simulink model "Simulation_in_Simulink"  (R2021b)
settings: Solver=FixedStepAuto  StartTime=0.0  StopTime=10  FixedStep=0.02  RelTol=1e-3
(part 5 of 5)

== matlab function Simulation_in_Simulink/M ==
  data: theta input; M output
function M = fcn(theta)


t1=theta(1);
t2=theta(2);
t3=theta(3);
t4=theta(4);
t5=theta(5);
t6=theta(6);


a2=0.6129;
a3=0.5716; 
d4=0.16389; 
d5=0.1157; 
d6=0.0922;

M = [(49450651*cos(2*t2 + 2*t3 + 2*t4 - t5))/250000000000 - (37373*d5)/2500000 - (37373*d4)/1250000 - (1966511423*cos(2*t2 + 2*t3 + 2*t4 - 2*t5))/20000000000000 - (1966511423*cos(2*t2 + 2*t3 + 2*t4 + 2*t5))/20000000000000 + (53*cos(2*t2))/40 + (1966511423*cos(2*t5))/10000000000000 - (3534581023*cos(2*t2 + 2*t3 + 2*t4))/10000000000000 + (42783*cos(2*t2 + 2*t3))/62500 - (49450651*cos(2*t2 + 2*t3 + 2*t4 + t5))/250000000000 + (37373*d5*cos(2*t2 + 2*t3 + 2*t4))/2500000 - (957929*a2*sin(2*t2 + t3 + t4 - t5))/100000000 + (957929*a3*sin(2*t2 + 2*t3 + t4 + t5))/100000000 + (sin(t2 + t3 + t4)^2*sin(t5)^2)/2500 - (210469*a2*sin(2*t2 + t3 + t4))/50000000 - (957929*a2*sin(t3 + t4 - t5))/100000000 + (8247*a2^2*cos(2*t2))/1000 - (1967*d5^2*cos(2*t2 + 2*t3 + 2*t4))/2000 + (cos(t2 + t3 + t4)*cos(t6) - sin(t2 + t3 + t4)*cos(t5)*sin(t6))*((3*cos(t2 + t3 + t4)*cos(t6))/12500 - (3*sin(t2 + t3 + t4)*cos(t5)*sin(t6))/12500) + (cos(t2 + t3 + t4)*sin(t6) + sin(t2 + t3 + t4)*cos(t5)*cos(t6))*((11*cos(t2 + t3 + t4)*sin(t6))/50000 + (11*sin(t2 + t3 + t4)*cos(t5)*cos(t6))/50000) + (957929*d5*cos(2*t2 + 2*t3 + 2*t4 + t5))/100000000 - (210469*a2*sin(t3 + t4))/50000000 + (957929*a3*sin(t4 + t5))/100000000 - (957929*a3*sin(2*t2 + 2*t3 + t4 - t5))/100000000 + (1967*a3^2*cos(2*t2 + 2*t3))/1000 + (2041*a2*cos(t3))/625 + (957929*d4*cos(t5))/25000000 + (d6*(cos(t5)*sin(t1) + cos(t2 + t3 + t4)*cos(t1)*sin(t5)) - (873*cos(t5)*sin(t1))/50000 - (19*sin(t6)*(sin(t1)*sin(t5) - cos(t2 + t3 + t4)*cos(t1)*cos(t5)))/20000 + d4*sin(t1) - (873*cos(t2 + t3 + t4)*cos(t1)*sin(t5))/50000 + (19*sin(t2 + t3 + t4)*cos(t1)*cos(t6))/20000 + a3*cos(t2 + t3)*cos(t1) + a2*cos(t1)*cos(t2) - d5*sin(t2 + t3 + t4)*cos(t1))*((43*d6*(cos(t5)*sin(t1) + cos(t2 + t3 + t4)*cos(t1)*sin(t5)))/100 - (37539*cos(t5)*sin(t1))/5000000 - (817*sin(t6)*(sin(t1)*sin(t5) - cos(t2 + t3 + t4)*cos(t1)*cos(t5)))/2000000 + (43*d4*sin(t1))/100 - (37539*cos(t2 + t3 + t4)*cos(t1)*sin(t5))/5000000 + (817*sin(t2 + t3 + t4)*cos(t1)*cos(t6))/2000000 + (43*a3*cos(t2 + t3)*cos(t1))/100 + (43*a2*cos(t1)*cos(t2))/100 - (43*d5*sin(t2 + t3 + t4)*cos(t1))/100) - (210469*a3*sin(t4))/50000000 - (210469*a3*sin(2*t2 + 2*t3 + t4))/50000000 + (8247*a2^2)/1000 + (1967*a3^2)/1000 + (957929*a2*sin(2*t2 + t3 + t4 + t5))/100000000 + (1967*d4^2)/500 + (1967*d5^2)/2000 + (2041*a2*cos(2*t2 + t3))/625 - (957929*d5*cos(2*t2 + 2*t3 + 2*t4 - t5))/100000000 - (957929*a3*sin(t4 - t5))/100000000 + (957929*a2*sin(t3 + t4 + t5))/100000000 + ((19*sin(t6)*(cos(t1)*sin(t5) + cos(t2 + t3 + t4)*cos(t5)*sin(t1)))/20000 + (873*cos(t1)*cos(t5))/50000 - d6*(cos(t1)*cos(t5) - cos(t2 + t3 + t4)*sin(t1)*sin(t5)) - d4*cos(t1) - (873*cos(t2 + t3 + t4)*sin(t1)*sin(t5))/50000 + (19*sin(t2 + t3 + t4)*cos(t6)*sin(t1))/20000 + a3*cos(t2 + t3)*sin(t1) + a2*cos(t2)*sin(t1) - d5*sin(t2 + t3 + t4)*sin(t1))*((817*sin(t6)*(cos(t1)*sin(t5) + cos(t2 + t3 + t4)*cos(t5)*sin(t1)))/2000000 + (37539*cos(t1)*cos(t5))/5000000 - (43*d6*(cos(t1)*cos(t5) - cos(t2 + t3 + t4)*sin(t1)*sin(t5)))/100 - (43*d4*cos(t1))/100 - (37539*cos(t2 + t3 + t4)*sin(t1)*sin(t5))/5000000 + (817*sin(t2 + t3 + t4)*cos(t6)*sin(t1))/2000000 + (43*a3*cos(t2 + t3)*sin(t1))/100 + (43*a2*cos(t2)*sin(t1))/100 - (43*d5*sin(t2 + t3 + t4)*sin(t1))/100) - (1967*a3*d5*sin(t4))/1000 - (1967*a3*d5*sin(2*t2 + 2*t3 + t4))/1000 + (1967*a2*a3*cos(2*t2 + t3))/500 - (1967*a2*d5*sin(2*t2 + t3 + t4))/1000 - (1967*a2*d5*sin(t3 + t4))/1000 + (1967*a2*a3*cos(t3))/500 + 5654679353183/2000000000000, (49450651*cos(t2 + t3 + t4))/125000000000 - (713241*cos(t2 + t3 + t4 + t5 + t6))/400000000000 - (713241*cos(t2 + t3 + t4 + t5 - t6))/400000000000 - (713241*cos(t2 + t3 + t4 - t5 + t6))/400000000000 + (784477*cos(t2 + t3 + t4 + t5 - 2*t6))/320000000000 - (784477*cos(t2 + t3 + t4 + t5 + 2*t6))/320000000000 - (713241*cos(t2 + t3 + t4 - 2*t5 + t6))/400000000000 - (713241*cos(t2 + t3 + t4 + 2*t5 + t6))/400000000000 + (49450651*cos(t2 + t3 + t4 + t5))/250000000000 - (2041*sin(t2 + t3))/12500 - (713241*cos(t2 + t3 + t4 - t5 - t6))/400000000000 - (784477*cos(t2 + t3 + t4 - t5 - 2*t6))/320000000000 + (784477*cos(t2 + t3 + t4 - t5 + 2*t6))/320000000000 + (713241*cos(t2 + t3 + t4 - 2*t5 - t6))/400000000000 + (713241*cos(t2 + t3 + t4 + 2*t5 - t6))/400000000000 + (784477*cos(t2 + t3 + t4 - 2*t5 - 2*t6))/640000000000 + (784477*cos(t2 + t3 + t4 - 2*t5 + 2*t6))/640000000000 - (784477*cos(t2 + t3 + t4 + 2*t5 - 2*t6))/640000000000 - (784477*cos(t2 + t3 + t4 + 2*t5 + 2*t6))/640000000000 - (1237*sin(t2))/1250 + (49450651*cos(t2 + t3 + t4 - t5))/250000000000 - (7474967197*cos(t2 + t3 + t4 - 2*t5))/40000000000000 + (7474967197*cos(t2 + t3 + t4 + 2*t5))/40000000000000 - (43*d6^2*cos(t2 + t3 + t4 - 2*t5))/400 + (43*d6^2*cos(t2 + t3 + t4 + 2*t5))/400 - (817*a3*sin(t2 + t3 - t5 - t6))/8000000 - (817*d4*cos(t2 + t3 + t4 + t5 - t6))/8000000 + (817*d4*cos(t2 + t3 + t4 - t5 + t6))/8000000 + (817*d5*cos(t2 + t3 + t4 + t5 - t6))/8000000 + (817*d5*cos(t2 + t3 + t4 - t5 + t6))/8000000 + (817*d6*cos(t2 + t3 + t4 + t5 - t6))/8000000 + (817*d6*cos(t2 + t3 + t4 - t5 + t6))/8000000 + (817*d6*cos(t2 + t3 + t4 - 2*t5 + t6))/8000000 + (817*d6*cos(t2 + t3 + t4 + 2*t5 + t6))/8000000 - (582539*a3*sin(t2 + t3 - t5))/100000000 + (817*a2*sin(t2 + t5 - t6))/8000000 + (817*a2*sin(t2 - t5 + t6))/8000000 + (817*a2*sin(t5 - t2 + t6))/8000000 + (582539*d4*cos(t2 + t3 + t4 + t5))/100000000 + (817*d4*cos(t2 + t3 + t4 + t6))/4000000 - (582539*d5*cos(t2 + t3 + t4 + t5))/100000000 - (817*a3*sin(t2 + t3 + t5 + t6))/8000000 + (37373*a3*sin(t2 + t3))/2500000 - (582539*a2*sin(t2 + t5))/100000000 - (817*d4*cos(t2 + t3 + t4 - t5 - t6))/8000000 - (817*d5*cos(t2 + t3 + t4 - t5 - t6))/8000000 + (817*d6*cos(t2 + t3 + t4 - t5 - t6))/8000000 - (817*d6*cos(t2 + t3 + t4 - 2*t5 - t6))/8000000 - (817*d6*cos(t2 + t3 + t4 + 2*t5 - t6))/8000000 - (1532627*a2*sin(t2))/2500000 - (582539*d4*cos(t2 + t3 + t4 - t5))/100000000 + (817*d4*cos(t2 + t3 + t4 - t6))/4000000 - (582539*d5*cos(t2 + t3 + t4 - t5))/100000000 + (37539*d6*cos(t2 + t3 + t4 - 2*t5))/10000000 - (37539*d6*cos(t2 + t3 + t4 + 2*t5))/10000000 + (817*a3*sin(t2 + t3 + t5 - t6))/8000000 + (817*a3*sin(t2 + t3 - t5 + t6))/8000000 + (817*d4*cos(t2 + t3 + t4 + t5 + t6))/8000000 - (817*d5*cos(t2 + t3 + t4 + t5 + t6))/8000000 + (817*d6*cos(t2 + t3 + t4 + t5 + t6))/8000000 - (582539*a2*sin(t2 - t5))/100000000 - (210469*d4*cos(t2 + t3 + t4))/50000000 - (582539*a3*sin(t2 + t3 + t5))/100000000 - (817*a2*sin(t2 + t5 + t6))/8000000 - (1091*a2*d4*sin(t2))/250 - (43*d4*d6*cos(t2 + t3 + t4 - t5))/200 - (43*d5*d6*cos(t2 + t3 + t4 - t5))/200 - (43*a2*d6*sin(t2 - t5))/200 - (2397*d4*d5*cos(t2 + t3 + t4))/1000 - (43*a3*d6*sin(t2 + t3 + t5))/200 - (43*a3*d6*sin(t2 + t3 - t5))/200 + (43*d4*d6*cos(t2 + t3 + t4 + t5))/200 - (43*d5*d6*cos(t2 + t3 + t4 + t5))/200 - (1091*a3*d4*sin(t2 + t3))/250 - (43*a2*d6*sin(t2 + t5))/200, (49450651*cos(t2 + t3 + t4))/125000000000 - (713241*cos(t2 + t3 + t4 + t5 + t6))/400000000000 - (713241*cos(t2 + t3 + t4 + t5 - t6))/400000000000 - (713241*cos(t2 + t3 + t4 - t5 + t6))/400000000000 + (784477*cos(t2 + t3 + t4 + t5 - 2*t6))/320000000000 - (784477*cos(t2 + t3 + t4 + t5 + 2*t6))/320000000000 - (713241*cos(t2 + t3 + t4 - 2*t5 + t6))/400000000000 - (713241*cos(t2 + t3 + t4 + 2*t5 + t6))/400000000000 + (49450651*cos(t2 + t3 + t4 + t5))/250000000000 - (2041*sin(t2 + t3))/12500 - (713241*cos(t2 + t3 + t4 - t5 - t6))/400000000000 - (784477*cos(t2 + t3 + t4 - t5 - 2*t6))/320000000000 + (784477*cos(t2 + t3 + t4 - t5 + 2*t6))/320000000000 + (713241*cos(t2 + t3 + t4 - 2*t5 - t6))/400000000000 + (713241*cos(t2 + t3 + t4 + 2*t5 - t6))/400000000000 + (784477*cos(t2 + t3 + t4 - 2*t5 - 2*t6))/640000000000 + (784477*cos(t2 + t3 + t4 - 2*t5 + 2*t6))/640000000000 - (784477*cos(t2 + t3 + t4 + 2*t5 - 2*t6))/640000000000 - (784477*cos(t2 + t3 + t4 + 2*t5 + 2*t6))/640000000000 + (49450651*cos(t2 + t3 + t4 - t5))/250000000000 - (7474967197*cos(t2 + t3 + t4 - 2*t5))/40000000000000 + (7474967197*cos(t2 + t3 + t4 + 2*t5))/40000000000000 - (43*d6^2*cos(t2 + t3 + t4 - 2*t5))/400 + (43*d6^2*cos(t2 + t3 + t4 + 2*t5))/400 - (817*a3*sin(t2 + t3 - t5 - t6))/8000000 - (817*d4*cos(t2 + t3 + t4 + t5 - t6))/8000000 + (817*d4*cos(t2 + t3 + t4 - t5 + t6))/8000000 + (817*d5*cos(t2 + t3 + t4 + t5 - t6))/8000000 + (817*d5*cos(t2 + t3 + t4 - t5 + t6))/8000000 + (817*d6*cos(t2 + t3 + t4 + t5 - t6))/8000000 + (817*d6*cos(t2 + t3 + t4 - t5 + t6))/8000000 + (817*d6*cos(t2 + t3 + t4 - 2*t5 + t6))/8000000 + (817*d6*cos(t2 + t3 + t4 + 2*t5 + t6))/8000000 - (582539*a3*sin(t2 + t3 - t5))/100000000 + (582539*d4*cos(t2 + t3 + t4 + t5))/100000000 + (817*d4*cos(t2 + t3 + t4 + t6))/4000000 - (582539*d5*cos(t2 + t3 + t4 + t5))/100000000 - (817*a3*sin(t2 + t3 + t5 + t6))/8000000 + (37373*a3*sin(t2 + t3))/2500000 - (817*d4*cos(t2 + t3 + t4 - t5 - t6))/8000000 - (817*d5*cos(t2 + t3 + t4 - t5 - t6))/8000000 + (817*d6*cos(t2 + t3 + t4 - t5 - t6))/8000000 - (817*d6*cos(t2 + t3 + t4 - 2*t5 - t6))/8000000 - (817*d6*cos(t2 + t3 + t4 + 2*t5 - t6))/8000000 - (582539*d4*cos(t2 + t3 + t4 - t5))/100000000 + (817*d4*cos(t2 + t3 + t4 - t6))/4000000 - (582539*d5*cos(t2 + t3 + t4 - t5))/100000000 + (37539*d6*cos(t2 + t3 + t4 - 2*t5))/10000000 - (37539*d6*cos(t2 + t3 + t4 + 2*t5))/10000000 + (817*a3*sin(t2 + t3 + t5 - t6))/8000000 + (817*a3*sin(t2 + t3 - t5 + t6))/8000000 + (817*d4*cos(t2 + t3 + t4 + t5 + t6))/8000000 - (817*d5*cos(t2 + t3 + t4 + t5 + t6))/8000000 + (817*d6*cos(t2 + t3 + t4 + t5 + t6))/8000000 - (210469*d4*cos(t2 + t3 + t4))/50000000 - (582539*a3*sin(t2 + t3 + t5))/100000000 - (43*d4*d6*cos(t2 + t3 + t4 - t5))/200 - (43*d5*d6*cos(t2 + t3 + t4 - t5))/200 - (2397*d4*d5*cos(t2 + t3 + t4))/1000 - (43*a3*d6*sin(t2 + t3 + t5))/200 - (43*a3*d6*sin(t2 + t3 - t5))/200 + (43*d4*d6*cos(t2 + t3 + t4 + t5))/200 - (43*d5*d6*cos(t2 + t3 + t4 + t5))/200 - (1091*a3*d4*sin(t2 + t3))/250, (49450651*cos(t2 + t3 + t4))/125000000000 - (713241*cos(t2 + t3 + t4 + t5 + t6))/400000000000 - (713241*cos(t2 + t3 + t4 + t5 - t6))/400000000000 - (713241*cos(t2 + t3 + t4 - t5 + t6))/400000000000 + (784477*cos(t2 + t3 + t4 + t5 - 2*t6))/320000000000 - (784477*cos(t2 + t3 + t4 + t5 + 2*t6))/320000000000 - (713241*cos(t2 + t3 + t4 - 2*t5 + t6))/400000000000 - (713241*cos(t2 + t3 + t4 + 2*t5 + t6))/400000000000 + (49450651*cos(t2 + t3 + t4 + t5))/250000000000 - (713241*cos(t2 + t3 + t4 - t5 - t6))/400000000000 - (784477*cos(t2 + t3 + t4 - t5 - 2*t6))/320000000000 + (784477*cos(t2 + t3 + t4 - t5 + 2*t6))/320000000000 + (713241*cos(t2 + t3 + t4 - 2*t5 - t6))/400000000000 + (713241*cos(t2 + t3 + t4 + 2*t5 - t6))/400000000000 + (784477*cos(t2 + t3 + t4 - 2*t5 - 2*t6))/640000000000 + (784477*cos(t2 + t3 + t4 - 2*t5 + 2*t6))/640000000000 - (784477*cos(t2 + t3 + t4 + 2*t5 - 2*t6))/640000000000 - (784477*cos(t2 + t3 + t4 + 2*t5 + 2*t6))/640000000000 + (49450651*cos(t2 + t3 + t4 - t5))/250000000000 - (7474967197*cos(t2 + t3 + t4 - 2*t5))/40000000000000 + (7474967197*cos(t2 + t3 + t4 + 2*t5))/40000000000000 - (43*d6^2*cos(t2 + t3 + t4 - 2*t5))/400 + (43*d6^2*cos(t2 + t3 + t4 + 2*t5))/400 - (817*d4*cos(t2 + t3 + t4 + t5 - t6))/8000000 + (817*d4*cos(t2 + t3 + t4 - t5 + t6))/8000000 + (817*d5*cos(t2 + t3 + t4 + t5 - t6))/8000000 + (817*d5*cos(t2 + t3 + t4 - t5 + t6))/8000000 + (817*d6*cos(t2 + t3 + t4 + t5 - t6))/8000000 + (817*d6*cos(t2 + t3 + t4 - t5 + t6))/8000000 + (817*d6*cos(t2 + t3 + t4 - 2*t5 + t6))/8000000 + (817*d6*cos(t2 + t3 + t4 + 2*t5 + t6))/8000000 + (582539*d4*cos(t2 + t3 + t4 + t5))/100000000 + (817*d4*cos(t2 + t3 + t4 + t6))/4000000 - (582539*d5*cos(t2 + t3 + t4 + t5))/100000000 - (817*d4*cos(t2 + t3 + t4 - t5 - t6))/8000000 - (817*d5*cos(t2 + t3 + t4 - t5 - t6))/8000000 + (817*d6*cos(t2 + t3 + t4 - t5 - t6))/8000000 - (817*d6*cos(t2 + t3 + t4 - 2*t5 - t6))/8000000 - (817*d6*cos(t2 + t3 + t4 + 2*t5 - t6))/8000000 - (582539*d4*cos(t2 + t3 + t4 - t5))/100000000 + (817*d4*cos(t2 + t3 + t4 - t6))/4000000 - (582539*d5*cos(t2 + t3 + t4 - t5))/100000000 + (37539*d6*cos(t2 + t3 + t4 - 2*t5))/10000000 - (37539*d6*cos(t2 + t3 + t4 + 2*t5))/10000000 + (817*d4*cos(t2 + t3 + t4 + t5 + t6))/8000000 - (817*d5*cos(t2 + t3 + t4 + t5 + t6))/8000000 + (817*d6*cos(t2 + t3 + t4 + t5 + t6))/8000000 - (210469*d4*cos(t2 + t3 + t4))/50000000 - (43*d4*d6*cos(t2 + t3 + t4 - t5))/200 - (43*d5*d6*cos(t2 + t3 + t4 - t5))/200 - (2397*d4*d5*cos(t2 + t3 + t4))/1000 + (43*d4*d6*cos(t2 + t3 + t4 + t5))/200 - (43*d5*d6*cos(t2 + t3 + t4 + t5))/200, (713241*cos(t2 + t3 + t4 + t5 + t6))/400000000000 + (33478847947*cos(t2 + t3 + t4))/10000000000000 + (713241*cos(t2 + t3 + t4 + t5 - t6))/400000000000 - (713241*cos(t2 + t3 + t4 - t5 + t6))/400000000000 - (784477*cos(t2 + t3 + t4 + t5 - 2*t6))/320000000000 + (784477*cos(t2 + t3 + t4 + t5 + 2*t6))/320000000000 - (49450651*cos(t2 + t3 + t4 + t5))/250000000000 - (713241*cos(t2 + t3 + t4 - t5 - t6))/400000000000 - (784477*cos(t2 + t3 + t4 - t5 - 2*t6))/320000000000 + (784477*cos(t2 + t3 + t4 - t5 + 2*t6))/320000000000 + (49450651*cos(t2 + t3 + t4 - t5))/250000000000 + (784477*cos(t2 + t3 + t4 - 2*t6))/160000000000 + (784477*cos(t2 + t3 + t4 + 2*t6))/160000000000 - (817*a3*sin(t2 + t3 - t5 - t6))/8000000 - (817*d4*cos(t2 + t3 + t4 + t5 - t6))/8000000 - (817*d4*cos(t2 + t3 + t4 - t5 + t6))/8000000 - (817*d5*cos(t2 + t3 + t4 + t5 - t6))/8000000 + (817*d5*cos(t2 + t3 + t4 - t5 + t6))/8000000 - (817*d6*cos(t2 + t3 + t4 + t5 - t6))/8000000 + (817*d6*cos(t2 + t3 + t4 - t5 + t6))/8000000 + (43*d6^2*cos(t2 + t3 + t4))/100 - (582539*a3*sin(t2 + t3 - t5))/100000000 - (817*a2*sin(t2 + t5 - t6))/8000000 + (817*a2*sin(t2 - t5 + t6))/8000000 + (817*a2*sin(t5 - t2 + t6))/8000000 + (582539*d4*cos(t2 + t3 + t4 + t5))/100000000 + (582539*d5*cos(t2 + t3 + t4 + t5))/100000000 + (817*a3*sin(t2 + t3 + t5 + t6))/8000000 + (582539*a2*sin(t2 + t5))/100000000 + (817*d4*cos(t2 + t3 + t4 - t5 - t6))/8000000 - (817*d5*cos(t2 + t3 + t4 - t5 - t6))/8000000 + (817*d6*cos(t2 + t3 + t4 - t5 - t6))/8000000 + (582539*d4*cos(t2 + t3 + t4 - t5))/100000000 - (582539*d5*cos(t2 + t3 + t4 - t5))/100000000 - (817*a3*sin(t2 + t3 + t5 - t6))/8000000 + (817*a3*sin(t2 + t3 - t5 + t6))/8000000 + (817*d4*cos(t2 + t3 + t4 + t5 + t6))/8000000 + (817*d5*cos(t2 + t3 + t4 + t5 + t6))/8000000 - (817*d6*cos(t2 + t3 + t4 + t5 + t6))/8000000 - (582539*a2*sin(t2 - t5))/100000000 - (37539*d6*cos(t2 + t3 + t4))/2500000 + (582539*a3*sin(t2 + t3 + t5))/100000000 + (817*a2*sin(t2 + t5 + t6))/8000000 + (43*d4*d6*cos(t2 + t3 + t4 - t5))/200 - (43*d5*d6*cos(t2 + t3 + t4 - t5))/200 - (43*a2*d6*sin(t2 - t5))/200 + (43*a3*d6*sin(t2 + t3 + t5))/200 - (43*a3*d6*sin(t2 + t3 - t5))/200 + (43*d4*d6*cos(t2 + t3 + t4 + t5))/200 + (43*d5*d6*cos(t2 + t3 + t4 + t5))/200 + (43*a2*d6*sin(t2 + t5))/200, (817*a2*cos(t2)*cos(t6)*sin(t5))/2000000 - (713241*cos(t2)*cos(t3)*cos(t4)*cos(t6))/100000000000 + (16015523*cos(t2)*cos(t3)*sin(t4)*sin(t5))/40000000000 + (16015523*cos(t2)*cos(t4)*sin(t3)*sin(t5))/40000000000 + (16015523*cos(t3)*cos(t4)*sin(t2)*sin(t5))/40000000000 + (713241*cos(t2)*cos(t6)*sin(t3)*sin(t4))/100000000000 + (713241*cos(t3)*cos(t6)*sin(t2)*sin(t4))/100000000000 + (713241*cos(t4)*cos(t6)*sin(t2)*sin(t3))/100000000000 - (16015523*sin(t2)*sin(t3)*sin(t4)*sin(t5))/40000000000 + (817*d6*cos(t2)*cos(t3)*cos(t4)*cos(t6))/2000000 + (817*a3*cos(t2)*cos(t3)*cos(t6)*sin(t5))/2000000 - (817*d4*cos(t2)*cos(t3)*sin(t4)*sin(t6))/2000000 - (817*d4*cos(t2)*cos(t4)*sin(t3)*sin(t6))/2000000 - (817*d4*cos(t3)*cos(t4)*sin(t2)*sin(t6))/2000000 - (817*d6*cos(t2)*cos(t6)*sin(t3)*sin(t4))/2000000 - (817*d6*cos(t3)*cos(t6)*sin(t2)*sin(t4))/2000000 - (817*d6*cos(t4)*cos(t6)*sin(t2)*sin(t3))/2000000 - (817*a3*cos(t6)*sin(t2)*sin(t3)*sin(t5))/2000000 + (817*d4*sin(t2)*sin(t3)*sin(t4)*sin(t6))/2000000 + (713241*cos(t2)*cos(t3)*cos(t5)*sin(t4)*sin(t6))/100000000000 + (713241*cos(t2)*cos(t4)*cos(t5)*sin(t3)*sin(t6))/100000000000 + (713241*cos(t3)*cos(t4)*cos(t5)*sin(t2)*sin(t6))/100000000000 - (713241*cos(t5)*sin(t2)*sin(t3)*sin(t4)*sin(t6))/100000000000 - (817*d4*cos(t2)*cos(t5)*cos(t6)*sin(t3)*sin(t4))/2000000 - (817*d4*cos(t3)*cos(t5)*cos(t6)*sin(t2)*sin(t4))/2000000 - (817*d4*cos(t4)*cos(t5)*cos(t6)*sin(t2)*sin(t3))/2000000 - (817*d5*cos(t2)*cos(t3)*cos(t6)*sin(t4)*sin(t5))/2000000 - (817*d5*cos(t2)*cos(t4)*cos(t6)*sin(t3)*sin(t5))/2000000 - (817*d5*cos(t3)*cos(t4)*cos(t6)*sin(t2)*sin(t5))/2000000 - (817*d6*cos(t2)*cos(t3)*cos(t5)*sin(t4)*sin(t6))/2000000 - (817*d6*cos(t2)*cos(t4)*cos(t5)*sin(t3)*sin(t6))/2000000 - (817*d6*cos(t3)*cos(t4)*cos(t5)*sin(t2)*sin(t6))/2000000 + (817*d5*cos(t6)*sin(t2)*sin(t3)*sin(t4)*sin(t5))/2000000 + (817*d6*cos(t5)*sin(t2)*sin(t3)*sin(t4)*sin(t6))/2000000 + (817*d4*cos(t2)*cos(t3)*cos(t4)*cos(t5)*cos(t6))/2000000;
                                                                                                              (49450651*cos(t2 + t3 + t4))/125000000000 - (713241*cos(t2 + t3 + t4 + t5 + t6))/400000000000 - (713241*cos(t2 + t3 + t4 + t5 - t6))/400000000000 - (713241*cos(t2 + t3 + t4 - t5 + t6))/400000000000 + (784477*cos(t2 + t3 + t4 + t5 - 2*t6))/320000000000 - (784477*cos(t2 + t3 + t4 + t5 + 2*t6))/320000000000 - (713241*cos(t2 + t3 + t4 - 2*t5 + t6))/400000000000 - (713241*cos(t2 + t3 + t4 + 2*t5 + t6))/400000000000 + (49450651*cos(t2 + t3 + t4 + t5))/250000000000 - (2041*sin(t2 + t3))/12500 - (713241*cos(t2 + t3 + t4 - t5 - t6))/400000000000 - (784477*cos(t2 + t3 + t4 - t5 - 2*t6))/320000000000 + (784477*cos(t2 + t3 + t4 - t5 + 2*t6))/320000000000 + (713241*cos(t2 + t3 + t4 - 2*t5 - t6))/400000000000 + (713241*cos(t2 + t3 + t4 + 2*t5 - t6))/400000000000 + (784477*cos(t2 + t3 + t4 - 2*t5 - 2*t6))/640000000000 + (784477*cos(t2 + t3 + t4 - 2*t5 + 2*t6))/640000000000 - (784477*cos(t2 + t3 + t4 + 2*t5 - 2*t6))/640000000000 - (784477*cos(t2 + t3 + t4 + 2*t5 + 2*t6))/640000000000 - (1237*sin(t2))/1250 + (49450651*cos(t2 + t3 + t4 - t5))/250000000000 - (7474967197*cos(t2 + t3 + t4 - 2*t5))/40000000000000 + (7474967197*cos(t2 + t3 + t4 + 2*t5))/40000000000000 - (43*d6^2*cos(t2 + t3 + t4 - 2*t5))/400 + (43*d6^2*cos(t2 + t3 + t4 + 2*t5))/400 - (817*a3*sin(t2 + t3 - t5 - t6))/8000000 - (817*d4*cos(t2 + t3 + t4 + t5 - t6))/8000000 + (817*d4*cos(t2 + t3 + t4 - t5 + t6))/8000000 + (817*d5*cos(t2 + t3 + t4 + t5 - t6))/8000000 + (817*d5*cos(t2 + t3 + t4 - t5 + t6))/8000000 + (817*d6*cos(t2 + t3 + t4 + t5 - t6))/8000000 + (817*d6*cos(t2 + t3 + t4 - t5 + t6))/8000000 + (817*d6*cos(t2 + t3 + t4 - 2*t5 + t6))/8000000 + (817*d6*cos(t2 + t3 + t4 + 2*t5 + t6))/8000000 - (582539*a3*sin(t2 + t3 - t5))/100000000 + (817*a2*sin(t2 + t5 - t6))/8000000 + (817*a2*sin(t2 - t5 + t6))/8000000 + (817*a2*sin(t5 - t2 + t6))/8000000 + (582539*d4*cos(t2 + t3 + t4 + t5))/100000000 + (817*d4*cos(t2 + t3 + t4 + t6))/4000000 - (582539*d5*cos(t2 + t3 + t4 + t5))/100000000 - (817*a3*sin(t2 + t3 + t5 + t6))/8000000 + (37373*a3*sin(t2 + t3))/2500000 - (582539*a2*sin(t2 + t5))/100000000 - (817*d4*cos(t2 + t3 + t4 - t5 - t6))/8000000 - (817*d5*cos(t2 + t3 + t4 - t5 - t6))/8000000 + (817*d6*cos(t2 + t3 + t4 - t5 - t6))/8000000 - (817*d6*cos(t2 + t3 + t4 - 2*t5 - t6))/8000000 - (817*d6*cos(t2 + t3 + t4 + 2*t5 - t6))/8000000 - (1532627*a2*sin(t2))/2500000 - (582539*d4*cos(t2 + t3 + t4 - t5))/100000000 + (817*d4*cos(t2 + t3 + t4 - t6))/4000000 - (582539*d5*cos(t2 + t3 + t4 - t5))/100000000 + (37539*d6*cos(t2 + t3 + t4 - 2*t5))/10000000 - (37539*d6*cos(t2 + t3 + t4 + 2*t5))/10000000 + (817*a3*sin(t2 + t3 + t5 - t6))/8000000 + (817*a3*sin(t2 + t3 - t5 + t6))/8000000 + (817*d4*cos(t2 + t3 + t4 + t5 + t6))/8000000 - (817*d5*cos(t2 + t3 + t4 + t5 + t6))/8000000 + (817*d6*cos(t2 + t3 + t4 + t5 + t6))/8000000 - (582539*a2*sin(t2 - t5))/100000000 - (210469*d4*cos(t2 + t3 + t4))/50000000 - (582539*a3*sin(t2 + t3 + t5))/100000000 - (817*a2*sin(t2 + t5 + t6))/8000000 - (1091*a2*d4*sin(t2))/250 - (43*d4*d6*cos(t2 + t3 + t4 - t5))/200 - (43*d5*d6*cos(t2 + t3 + t4 - t5))/200 - (43*a2*d6*sin(t2 - t5))/200 - (2397*d4*d5*cos(t2 + t3 + t4))/1000 - (43*a3*d6*sin(t2 + t3 + t5))/200 - (43*a3*d6*sin(t2 + t3 - t5))/200 + (43*d4*d6*cos(t2 + t3 + t4 + t5))/200 - (43*d5*d6*cos(t2 + t3 + t4 + t5))/200 - (1091*a3*d4*sin(t2 + t3))/250 - (43*a2*d6*sin(t2 + t5))/200,                                                                                                                                                                                                                                                                                                                                                                                                                                                                                                                                                                                                                                                                                                                                                                                                                                                                                                                                                                                                                                                                                                                                                                                                                                                                                                                                                                                                                                                                                                                                                                                                                                                                                                                                                                                                                                                                                                                                                                                                                                                                                                                                                                                                                               (4082*a2*cos(t3))/625 - (37539*d6)/2500000 - (3786513411*cos(t5)^2)/5000000000000 - (784477*cos(t6)^2)/40000000000 - (43*d6^2*cos(t5)^2)/100 - (37373*d5)/1250000 - (817*d5*cos(t6))/1000000 - (210469*a3*sin(t4))/25000000 + (4231*a2^2)/250 + (1091*a3^2)/250 + (2397*d5^2)/1000 + (43*d6^2)/100 + (784477*cos(t5)^2*cos(t6)^2)/40000000000 + (37539*d6*cos(t5)^2)/2500000 - (713241*cos(t5)*sin(t5)*sin(t6))/50000000000 - (2397*a3*d5*sin(t4))/500 - (210469*a2*cos(t3)*sin(t4))/25000000 - (210469*a2*cos(t4)*sin(t3))/25000000 + (582539*a3*cos(t4)*sin(t5))/25000000 + (817*a3*cos(t6)*sin(t4))/1000000 + (1091*a2*a3*cos(t3))/125 + (582539*a2*cos(t3)*cos(t4)*sin(t5))/25000000 + (817*a2*cos(t3)*cos(t6)*sin(t4))/1000000 + (817*a2*cos(t4)*cos(t6)*sin(t3))/1000000 + (817*a3*cos(t4)*cos(t5)*sin(t6))/1000000 + (817*d6*cos(t5)*sin(t5)*sin(t6))/1000000 - (582539*a2*sin(t3)*sin(t4)*sin(t5))/25000000 - (2397*a2*d5*cos(t3)*sin(t4))/500 - (2397*a2*d5*cos(t4)*sin(t3))/500 + (43*a3*d6*cos(t4)*sin(t5))/50 + (817*a2*cos(t3)*cos(t4)*cos(t5)*sin(t6))/1000000 - (817*a2*cos(t5)*sin(t3)*sin(t4)*sin(t6))/1000000 + (43*a2*d6*cos(t3)*cos(t4)*sin(t5))/50 - (43*a2*d6*sin(t3)*sin(t4)*sin(t5))/50 + 2553571193279/625000000000,                                                                                                                                                                                                                                                                                                                                                                                                                                                                                                                                                                                                                                                                                                                                                                                                                                                                                                                                                                                                                                                                                                                                                                                                                                                                                                                                                                                                                                                                                                                                                                                                                                                                                                                                                                                                                                                                    (2041*a2*cos(t3))/625 - (37539*d6)/2500000 - (3786513411*cos(t5)^2)/5000000000000 - (784477*cos(t6)^2)/40000000000 - (43*d6^2*cos(t5)^2)/100 - (37373*d5)/1250000 - (817*d5*cos(t6))/1000000 - (210469*a3*sin(t4))/25000000 + (1091*a3^2)/250 + (2397*d5^2)/1000 + (43*d6^2)/100 + (784477*cos(t5)^2*cos(t6)^2)/40000000000 + (37539*d6*cos(t5)^2)/2500000 - (713241*cos(t5)*sin(t5)*sin(t6))/50000000000 - (2397*a3*d5*sin(t4))/500 - (210469*a2*cos(t3)*sin(t4))/50000000 - (210469*a2*cos(t4)*sin(t3))/50000000 + (582539*a3*cos(t4)*sin(t5))/25000000 + (817*a3*cos(t6)*sin(t4))/1000000 + (1091*a2*a3*cos(t3))/250 + (582539*a2*cos(t3)*cos(t4)*sin(t5))/50000000 + (817*a2*cos(t3)*cos(t6)*sin(t4))/2000000 + (817*a2*cos(t4)*cos(t6)*sin(t3))/2000000 + (817*a3*cos(t4)*cos(t5)*sin(t6))/1000000 + (817*d6*cos(t5)*sin(t5)*sin(t6))/1000000 - (582539*a2*sin(t3)*sin(t4)*sin(t5))/50000000 - (2397*a2*d5*cos(t3)*sin(t4))/1000 - (2397*a2*d5*cos(t4)*sin(t3))/1000 + (43*a3*d6*cos(t4)*sin(t5))/50 + (817*a2*cos(t3)*cos(t4)*cos(t5)*sin(t6))/2000000 - (817*a2*cos(t5)*sin(t3)*sin(t4)*sin(t6))/2000000 + (43*a2*d6*cos(t3)*cos(t4)*sin(t5))/100 - (43*a2*d6*sin(t3)*sin(t4)*sin(t5))/100 + 872321193279/625000000000,                                                                                                                                                                                                                                                                                                                                                                                                                                                                                                                                                                                                                                                                                                                                                                                                                                                                                                                                                                                                                                                                                                                                                                                                                                                                                                                                                                                                                                                                                                         (2397*d5^2)/1000 - (37539*d6)/2500000 - (3786513411*cos(t5)^2)/5000000000000 - (784477*cos(t6)^2)/40000000000 - (43*d6^2*cos(t5)^2)/100 - (817*d5*cos(t6))/1000000 - (210469*a3*sin(t4))/50000000 - (37373*d5)/1250000 + (43*d6^2)/100 + (784477*cos(t5)^2*cos(t6)^2)/40000000000 + (37539*d6*cos(t5)^2)/2500000 - (713241*cos(t5)*sin(t5)*sin(t6))/50000000000 - (2397*a3*d5*sin(t4))/1000 - (210469*a2*cos(t3)*sin(t4))/50000000 - (210469*a2*cos(t4)*sin(t3))/50000000 + (582539*a3*cos(t4)*sin(t5))/50000000 + (817*a3*cos(t6)*sin(t4))/2000000 + (582539*a2*cos(t3)*cos(t4)*sin(t5))/50000000 + (817*a2*cos(t3)*cos(t6)*sin(t4))/2000000 + (817*a2*cos(t4)*cos(t6)*sin(t3))/2000000 + (817*a3*cos(t4)*cos(t5)*sin(t6))/2000000 + (817*d6*cos(t5)*sin(t5)*sin(t6))/1000000 - (582539*a2*sin(t3)*sin(t4)*sin(t5))/50000000 - (2397*a2*d5*cos(t3)*sin(t4))/1000 - (2397*a2*d5*cos(t4)*sin(t3))/1000 + (43*a3*d6*cos(t4)*sin(t5))/100 + (817*a2*cos(t3)*cos(t4)*cos(t5)*sin(t6))/2000000 - (817*a2*cos(t5)*sin(t3)*sin(t4)*sin(t6))/2000000 + (43*a2*d6*cos(t3)*cos(t4)*sin(t5))/100 - (43*a2*d6*sin(t3)*sin(t4)*sin(t5))/100 + 4161193279/625000000000,                                                                                                                                                                                                                                                                                                                                                                                                                                                                                                                                                                                                                                                                                                                                                                                                                                                                                                                                                                                                                                                                                                                                                                                                                                                                                                                                                                                                                                                                                                                                                                                                                                                                                   (49450651*cos(t5))/125000000000 - (713241*cos(t5)*cos(t6))/100000000000 - (582539*d5*cos(t5))/50000000 + (784477*cos(t6)*sin(t5)*sin(t6))/40000000000 + (817*d6*cos(t5)*cos(t6))/2000000 + (582539*a3*cos(t5)*sin(t4))/50000000 + (817*d5*sin(t5)*sin(t6))/2000000 - (43*d5*d6*cos(t5))/100 + (582539*a2*cos(t3)*cos(t5)*sin(t4))/50000000 + (582539*a2*cos(t4)*cos(t5)*sin(t3))/50000000 - (817*a3*sin(t4)*sin(t5)*sin(t6))/2000000 + (43*a3*d6*cos(t5)*sin(t4))/100 - (817*a2*cos(t3)*sin(t4)*sin(t5)*sin(t6))/2000000 - (817*a2*cos(t4)*sin(t3)*sin(t5)*sin(t6))/2000000 + (43*a2*d6*cos(t3)*cos(t5)*sin(t4))/100 + (43*a2*d6*cos(t4)*cos(t5)*sin(t3))/100,                                                                                                                                                                                                                                                                                                                                                                                                                                                                                                                                                                                                                                                                                                                                                                                                                                                                                                                                                                                                                                                                                                                                                                                                                                                                                                                                                                                                                                                                                                                                                                                                                         (16015523*cos(t5))/40000000000 - (713241*sin(t5)*sin(t6))/100000000000 - (817*d5*cos(t5)*cos(t6))/2000000 + (817*a3*cos(t4)*sin(t6))/2000000 + (817*d6*sin(t5)*sin(t6))/2000000 + (817*a2*cos(t3)*cos(t4)*sin(t6))/2000000 + (817*a3*cos(t5)*cos(t6)*sin(t4))/2000000 - (817*a2*sin(t3)*sin(t4)*sin(t6))/2000000 + (817*a2*cos(t3)*cos(t5)*cos(t6)*sin(t4))/2000000 + (817*a2*cos(t4)*cos(t5)*cos(t6)*sin(t3))/2000000;
                                                                                                                                                                                                                                                                                                                                                                                                                                                                                        (49450651*cos(t2 + t3 + t4))/125000000000 - (713241*cos(t2 + t3 + t4 + t5 + t6))/400000000000 - (713241*cos(t2 + t3 + t4 + t5 - t6))/400000000000 - (713241*cos(t2 + t3 + t4 - t5 + t6))/400000000000 + (784477*cos(t2 + t3 + t4 + t5 - 2*t6))/320000000000 - (784477*cos(t2 + t3 + t4 + t5 + 2*t6))/320000000000 - (713241*cos(t2 + t3 + t4 - 2*t5 + t6))/400000000000 - (713241*cos(t2 + t3 + t4 + 2*t5 + t6))/400000000000 + (49450651*cos(t2 + t3 + t4 + t5))/250000000000 - (2041*sin(t2 + t3))/12500 - (713241*cos(t2 + t3 + t4 - t5 - t6))/400000000000 - (784477*cos(t2 + t3 + t4 - t5 - 2*t6))/320000000000 + (784477*cos(t2 + t3 + t4 - t5 + 2*t6))/320000000000 + (713241*cos(t2 + t3 + t4 - 2*t5 - t6))/400000000000 + (713241*cos(t2 + t3 + t4 + 2*t5 - t6))/400000000000 + (784477*cos(t2 + t3 + t4 - 2*t5 - 2*t6))/640000000000 + (784477*cos(t2 + t3 + t4 - 2*t5 + 2*t6))/640000000000 - (784477*cos(t2 + t3 + t4 + 2*t5 - 2*t6))/640000000000 - (784477*cos(t2 + t3 + t4 + 2*t5 + 2*t6))/640000000000 + (49450651*cos(t2 + t3 + t4 - t5))/250000000000 - (7474967197*cos(t2 + t3 + t4 - 2*t5))/40000000000000 + (7474967197*cos(t2 + t3 + t4 + 2*t5))/40000000000000 - (43*d6^2*cos(t2 + t3 + t4 - 2*t5))/400 + (43*d6^2*cos(t2 + t3 + t4 + 2*t5))/400 - (817*a3*sin(t2 + t3 - t5 - t6))/8000000 - (817*d4*cos(t2 + t3 + t4 + t5 - t6))/8000000 + (817*d4*cos(t2 + t3 + t4 - t5 + t6))/8000000 + (817*d5*cos(t2 + t3 + t4 + t5 - t6))/8000000 + (817*d5*cos(t2 + t3 + t4 - t5 + t6))/8000000 + (817*d6*cos(t2 + t3 + t4 + t5 - t6))/8000000 + (817*d6*cos(t2 + t3 + t4 - t5 + t6))/8000000 + (817*d6*cos(t2 + t3 + t4 - 2*t5 + t6))/8000000 + (817*d6*cos(t2 + t3 + t4 + 2*t5 + t6))/8000000 - (582539*a3*sin(t2 + t3 - t5))/100000000 + (582539*d4*cos(t2 + t3 + t4 + t5))/100000000 + (817*d4*cos(t2 + t3 + t4 + t6))/4000000 - (582539*d5*cos(t2 + t3 + t4 + t5))/100000000 - (817*a3*sin(t2 + t3 + t5 + t6))/8000000 + (37373*a3*sin(t2 + t3))/2500000 - (817*d4*cos(t2 + t3 + t4 - t5 - t6))/8000000 - (817*d5*cos(t2 + t3 + t4 - t5 - t6))/8000000 + (817*d6*cos(t2 + t3 + t4 - t5 - t6))/8000000 - (817*d6*cos(t2 + t3 + t4 - 2*t5 - t6))/8000000 - (817*d6*cos(t2 + t3 + t4 + 2*t5 - t6))/8000000 - (582539*d4*cos(t2 + t3 + t4 - t5))/100000000 + (817*d4*cos(t2 + t3 + t4 - t6))/4000000 - (582539*d5*cos(t2 + t3 + t4 - t5))/100000000 + (37539*d6*cos(t2 + t3 + t4 - 2*t5))/10000000 - (37539*d6*cos(t2 + t3 + t4 + 2*t5))/10000000 + (817*a3*sin(t2 + t3 + t5 - t6))/8000000 + (817*a3*sin(t2 + t3 - t5 + t6))/8000000 + (817*d4*cos(t2 + t3 + t4 + t5 + t6))/8000000 - (817*d5*cos(t2 + t3 + t4 + t5 + t6))/8000000 + (817*d6*cos(t2 + t3 + t4 + t5 + t6))/8000000 - (210469*d4*cos(t2 + t3 + t4))/50000000 - (582539*a3*sin(t2 + t3 + t5))/100000000 - (43*d4*d6*cos(t2 + t3 + t4 - t5))/200 - (43*d5*d6*cos(t2 + t3 + t4 - t5))/200 - (2397*d4*d5*cos(t2 + t3 + t4))/1000 - (43*a3*d6*sin(t2 + t3 + t5))/200 - (43*a3*d6*sin(t2 + t3 - t5))/200 + (43*d4*d6*cos(t2 + t3 + t4 + t5))/200 - (43*d5*d6*cos(t2 + t3 + t4 + t5))/200 - (1091*a3*d4*sin(t2 + t3))/250,                                                                                                                                                                                                                                                                                                                                                                                                                                                                                                                                                                                                                                                                                                                                                                                                                                                                                                                                                                                                                                                                                                                                                                                                                                                                                                                                                                                                                                                                                                                                                                                                                                                                                                                                                                                                                                                                                                                                                                                                                                                                                                                                                                                                                                              (2041*a2*cos(t3))/625 - (37539*d6)/2500000 - (3786513411*cos(t5)^2)/5000000000000 - (784477*cos(t6)^2)/40000000000 - (43*d6^2*cos(t5)^2)/100 - (37373*d5)/1250000 - (817*d5*cos(t6))/1000000 - (210469*a3*sin(t4))/25000000 + (1091*a3^2)/250 + (2397*d5^2)/1000 + (43*d6^2)/100 + (784477*cos(t5)^2*cos(t6)^2)/40000000000 + (37539*d6*cos(t5)^2)/2500000 - (713241*cos(t5)*sin(t5)*sin(t6))/50000000000 - (2397*a3*d5*sin(t4))/500 - (210469*a2*cos(t3)*sin(t4))/50000000 - (210469*a2*cos(t4)*sin(t3))/50000000 + (582539*a3*cos(t4)*sin(t5))/25000000 + (817*a3*cos(t6)*sin(t4))/1000000 + (1091*a2*a3*cos(t3))/250 + (582539*a2*cos(t3)*cos(t4)*sin(t5))/50000000 + (817*a2*cos(t3)*cos(t6)*sin(t4))/2000000 + (817*a2*cos(t4)*cos(t6)*sin(t3))/2000000 + (817*a3*cos(t4)*cos(t5)*sin(t6))/1000000 + (817*d6*cos(t5)*sin(t5)*sin(t6))/1000000 - (582539*a2*sin(t3)*sin(t4)*sin(t5))/50000000 - (2397*a2*d5*cos(t3)*sin(t4))/1000 - (2397*a2*d5*cos(t4)*sin(t3))/1000 + (43*a3*d6*cos(t4)*sin(t5))/50 + (817*a2*cos(t3)*cos(t4)*cos(t5)*sin(t6))/2000000 - (817*a2*cos(t5)*sin(t3)*sin(t4)*sin(t6))/2000000 + (43*a2*d6*cos(t3)*cos(t4)*sin(t5))/100 - (43*a2*d6*sin(t3)*sin(t4)*sin(t5))/100 + 872321193279/625000000000,                                                                                                                                                                                                                                                                                                                                                                                                                                                                                                                                                                                                                                                                                                                                                                                                                                                                                                                                                                                                                                                                                                                                                                                                                                                                                                                                                                                                                                                                                                                                                                                                                                                                                                                                                                                                                                                                                                                                                                                                                                                                                                                                                                                                                                                                                                                                                                                                                                                         (1091*a3^2)/250 - (37539*d6)/2500000 - (3786513411*cos(t5)^2)/5000000000000 - (784477*cos(t6)^2)/40000000000 - (43*d6^2*cos(t5)^2)/100 - (817*d5*cos(t6))/1000000 - (210469*a3*sin(t4))/25000000 - (37373*d5)/1250000 + (2397*d5^2)/1000 + (43*d6^2)/100 + (784477*cos(t5)^2*cos(t6)^2)/40000000000 + (37539*d6*cos(t5)^2)/2500000 - (713241*cos(t5)*sin(t5)*sin(t6))/50000000000 - (2397*a3*d5*sin(t4))/500 + (582539*a3*cos(t4)*sin(t5))/25000000 + (817*a3*cos(t6)*sin(t4))/1000000 + (817*a3*cos(t4)*cos(t5)*sin(t6))/1000000 + (817*d6*cos(t5)*sin(t5)*sin(t6))/1000000 + (43*a3*d6*cos(t4)*sin(t5))/50 + 872321193279/625000000000,                                                                                                                                                                                                                                                                                                                                                                                                                                                                                                                                                                                                                                                                                                                                                                                                                                                                                                                                                                                                                                                                                                                                                                                                                                                                                                                                                                                                                                                                                                                                                                                                                                                                                                                                                                                                                                                                                                                                                                                                                                           (2397*d5^2)/1000 - (37539*d6)/2500000 - (3786513411*cos(t5)^2)/5000000000000 - (784477*cos(t6)^2)/40000000000 - (43*d6^2*cos(t5)^2)/100 - (817*d5*cos(t6))/1000000 - (210469*a3*sin(t4))/50000000 - (37373*d5)/1250000 + (43*d6^2)/100 + (784477*cos(t5)^2*cos(t6)^2)/40000000000 + (37539*d6*cos(t5)^2)/2500000 - (713241*cos(t5)*sin(t5)*sin(t6))/50000000000 - (2397*a3*d5*sin(t4))/1000 + (582539*a3*cos(t4)*sin(t5))/50000000 + (817*a3*cos(t6)*sin(t4))/2000000 + (817*a3*cos(t4)*cos(t5)*sin(t6))/2000000 + (817*d6*cos(t5)*sin(t5)*sin(t6))/1000000 + (43*a3*d6*cos(t4)*sin(t5))/100 + 4161193279/625000000000,                                                                                                                                                                                                                                                                                                                                                                                                                                                                                                                                                                                                                                                                                                                                                                                                                                                                                                                                                                                                                                                                                                                                                                                                                                                                                                                                                                                                                                                                                                                                                                                                                                                                                                                                                                                                                                                                                                                                                                         (49450651*cos(t5))/125000000000 - (713241*cos(t5)*cos(t6))/100000000000 - (582539*d5*cos(t5))/50000000 + (784477*cos(t6)*sin(t5)*sin(t6))/40000000000 + (817*d6*cos(t5)*cos(t6))/2000000 + (582539*a3*cos(t5)*sin(t4))/50000000 + (817*d5*sin(t5)*sin(t6))/2000000 - (43*d5*d6*cos(t5))/100 - (817*a3*sin(t4)*sin(t5)*sin(t6))/2000000 + (43*a3*d6*cos(t5)*sin(t4))/100,                                                                                                                                                                                                                                                                                                                                                                                                                                                                                                                                                                                                                                                                                                                                                                                                                                                                                                                                                                                                                                                                                                                                                                                                                                                                                                                                                                                                                                                                                                                                                                                                                                                                                                                                                                                                                     (16015523*cos(t5))/40000000000 - (713241*sin(t5)*sin(t6))/100000000000 - (817*d5*cos(t5)*cos(t6))/2000000 + (817*a3*cos(t4)*sin(t6))/2000000 + (817*d6*sin(t5)*sin(t6))/2000000 + (817*a3*cos(t5)*cos(t6)*sin(t4))/2000000;
                                                                                                                                                                                                                                                                                                                                                                                                                                                                                                                                                                                                                                                                                                                                                                                                                                                                                                                        (49450651*cos(t2 + t3 + t4))/125000000000 - (713241*cos(t2 + t3 + t4 + t5 + t6))/400000000000 - (713241*cos(t2 + t3 + t4 + t5 - t6))/400000000000 - (713241*cos(t2 + t3 + t4 - t5 + t6))/400000000000 + (784477*cos(t2 + t3 + t4 + t5 - 2*t6))/320000000000 - (784477*cos(t2 + t3 + t4 + t5 + 2*t6))/320000000000 - (713241*cos(t2 + t3 + t4 - 2*t5 + t6))/400000000000 - (713241*cos(t2 + t3 + t4 + 2*t5 + t6))/400000000000 + (49450651*cos(t2 + t3 + t4 + t5))/250000000000 - (713241*cos(t2 + t3 + t4 - t5 - t6))/400000000000 - (784477*cos(t2 + t3 + t4 - t5 - 2*t6))/320000000000 + (784477*cos(t2 + t3 + t4 - t5 + 2*t6))/320000000000 + (713241*cos(t2 + t3 + t4 - 2*t5 - t6))/400000000000 + (713241*cos(t2 + t3 + t4 + 2*t5 - t6))/400000000000 + (784477*cos(t2 + t3 + t4 - 2*t5 - 2*t6))/640000000000 + (784477*cos(t2 + t3 + t4 - 2*t5 + 2*t6))/640000000000 - (784477*cos(t2 + t3 + t4 + 2*t5 - 2*t6))/640000000000 - (784477*cos(t2 + t3 + t4 + 2*t5 + 2*t6))/640000000000 + (49450651*cos(t2 + t3 + t4 - t5))/250000000000 - (7474967197*cos(t2 + t3 + t4 - 2*t5))/40000000000000 + (7474967197*cos(t2 + t3 + t4 + 2*t5))/40000000000000 - (43*d6^2*cos(t2 + t3 + t4 - 2*t5))/400 + (43*d6^2*cos(t2 + t3 + t4 + 2*t5))/400 - (817*d4*cos(t2 + t3 + t4 + t5 - t6))/8000000 + (817*d4*cos(t2 + t3 + t4 - t5 + t6))/8000000 + (817*d5*cos(t2 + t3 + t4 + t5 - t6))/8000000 + (817*d5*cos(t2 + t3 + t4 - t5 + t6))/8000000 + (817*d6*cos(t2 + t3 + t4 + t5 - t6))/8000000 + (817*d6*cos(t2 + t3 + t4 - t5 + t6))/8000000 + (817*d6*cos(t2 + t3 + t4 - 2*t5 + t6))/8000000 + (817*d6*cos(t2 + t3 + t4 + 2*t5 + t6))/8000000 + (582539*d4*cos(t2 + t3 + t4 + t5))/100000000 + (817*d4*cos(t2 + t3 + t4 + t6))/4000000 - (582539*d5*cos(t2 + t3 + t4 + t5))/100000000 - (817*d4*cos(t2 + t3 + t4 - t5 - t6))/8000000 - (817*d5*cos(t2 + t3 + t4 - t5 - t6))/8000000 + (817*d6*cos(t2 + t3 + t4 - t5 - t6))/8000000 - (817*d6*cos(t2 + t3 + t4 - 2*t5 - t6))/8000000 - (817*d6*cos(t2 + t3 + t4 + 2*t5 - t6))/8000000 - (582539*d4*cos(t2 + t3 + t4 - t5))/100000000 + (817*d4*cos(t2 + t3 + t4 - t6))/4000000 - (582539*d5*cos(t2 + t3 + t4 - t5))/100000000 + (37539*d6*cos(t2 + t3 + t4 - 2*t5))/10000000 - (37539*d6*cos(t2 + t3 + t4 + 2*t5))/10000000 + (817*d4*cos(t2 + t3 + t4 + t5 + t6))/8000000 - (817*d5*cos(t2 + t3 + t4 + t5 + t6))/8000000 + (817*d6*cos(t2 + t3 + t4 + t5 + t6))/8000000 - (210469*d4*cos(t2 + t3 + t4))/50000000 - (43*d4*d6*cos(t2 + t3 + t4 - t5))/200 - (43*d5*d6*cos(t2 + t3 + t4 - t5))/200 - (2397*d4*d5*cos(t2 + t3 + t4))/1000 + (43*d4*d6*cos(t2 + t3 + t4 + t5))/200 - (43*d5*d6*cos(t2 + t3 + t4 + t5))/200,                                                                                                                                                                                                                                                                                                                                                                                                                                                                                                                                                                                                                                                                                                                                                                                                                                                                                                                                                                                                                                                                                                                                                                                                                                                                                                                                                                                                                                                                                                                                                                                                                                                                                                                                                                                                                                                                                                                                                                                                                                                                                                                                                                                                                                                                                                                   (2397*d5^2)/1000 - (37539*d6)/2500000 - (3786513411*cos(t5)^2)/5000000000000 - (784477*cos(t6)^2)/40000000000 - (43*d6^2*cos(t5)^2)/100 - (817*d5*cos(t6))/1000000 - (210469*a3*sin(t4))/50000000 - (37373*d5)/1250000 + (43*d6^2)/100 + (784477*cos(t5)^2*cos(t6)^2)/40000000000 + (37539*d6*cos(t5)^2)/2500000 - (713241*cos(t5)*sin(t5)*sin(t6))/50000000000 - (2397*a3*d5*sin(t4))/1000 - (210469*a2*cos(t3)*sin(t4))/50000000 - (210469*a2*cos(t4)*sin(t3))/50000000 + (582539*a3*cos(t4)*sin(t5))/50000000 + (817*a3*cos(t6)*sin(t4))/2000000 + (582539*a2*cos(t3)*cos(t4)*sin(t5))/50000000 + (817*a2*cos(t3)*cos(t6)*sin(t4))/2000000 + (817*a2*cos(t4)*cos(t6)*sin(t3))/2000000 + (817*a3*cos(t4)*cos(t5)*sin(t6))/2000000 + (817*d6*cos(t5)*sin(t5)*sin(t6))/1000000 - (582539*a2*sin(t3)*sin(t4)*sin(t5))/50000000 - (2397*a2*d5*cos(t3)*sin(t4))/1000 - (2397*a2*d5*cos(t4)*sin(t3))/1000 + (43*a3*d6*cos(t4)*sin(t5))/100 + (817*a2*cos(t3)*cos(t4)*cos(t5)*sin(t6))/2000000 - (817*a2*cos(t5)*sin(t3)*sin(t4)*sin(t6))/2000000 + (43*a2*d6*cos(t3)*cos(t4)*sin(t5))/100 - (43*a2*d6*sin(t3)*sin(t4)*sin(t5))/100 + 4161193279/625000000000,                                                                                                                                                                                                                                                                                                                                                                                                                                                                                                                                                                                                                                                                                                                                                                                                                                                                                                                                                                                                                                                                                                                                                                                                                                                                                                                                                                                                                                                                                                                                                                                                                                                                                                                                                                                                                                                                                                                                                                                                                                                                                                                                                                                                                                                                                                                                                                                                                                                                           (2397*d5^2)/1000 - (37539*d6)/2500000 - (3786513411*cos(t5)^2)/5000000000000 - (784477*cos(t6)^2)/40000000000 - (43*d6^2*cos(t5)^2)/100 - (817*d5*cos(t6))/1000000 - (210469*a3*sin(t4))/50000000 - (37373*d5)/1250000 + (43*d6^2)/100 + (784477*cos(t5)^2*cos(t6)^2)/40000000000 + (37539*d6*cos(t5)^2)/2500000 - (713241*cos(t5)*sin(t5)*sin(t6))/50000000000 - (2397*a3*d5*sin(t4))/1000 + (582539*a3*cos(t4)*sin(t5))/50000000 + (817*a3*cos(t6)*sin(t4))/2000000 + (817*a3*cos(t4)*cos(t5)*sin(t6))/2000000 + (817*d6*cos(t5)*sin(t5)*sin(t6))/1000000 + (43*a3*d6*cos(t4)*sin(t5))/100 + 4161193279/625000000000,                                                                                                                                                                                                                                                                                                                                                                                                                                                                                                                                                                                                                                                                                                                                                                                                                                                                                                                                                                                                                                                                                                                                                                                                                                                                                                                                                                                                                                                                                                                                                                                                                                                                                                                                                                                                                                                                                                                                                                                                                                                                                                                                                                                                                                                            (2397*d5^2)/1000 - (37539*d6)/2500000 - (3786513411*cos(t5)^2)/5000000000000 - (784477*cos(t6)^2)/40000000000 - (43*d6^2*cos(t5)^2)/100 - (817*d5*cos(t6))/1000000 - (37373*d5)/1250000 + (43*d6^2)/100 + (784477*cos(t5)^2*cos(t6)^2)/40000000000 + (37539*d6*cos(t5)^2)/2500000 - (713241*cos(t5)*sin(t5)*sin(t6))/50000000000 + (817*d6*cos(t5)*sin(t5)*sin(t6))/1000000 + 4161193279/625000000000,                                                                                                                                                                                                                                                                                                                                                                                                                                                                                                                                                                                                                                                                                                                                                                                                                                                                                                                                                                                                                                                                                                                                                                                                                                                                                                                                                                                                                                                                                                                                                                                                                                                                                                                                                                                                                                                                                                                                                                                                                                                                                            (49450651*cos(t5))/125000000000 - (713241*cos(t5)*cos(t6))/100000000000 - (582539*d5*cos(t5))/50000000 + (784477*cos(t6)*sin(t5)*sin(t6))/40000000000 + (817*d6*cos(t5)*cos(t6))/2000000 + (817*d5*sin(t5)*sin(t6))/2000000 - (43*d5*d6*cos(t5))/100,                                                                                                                                                                                                                                                                                                                                                                                                                                                                                                                                                                                                                                                                                                                                                                                                                                                                                                                                                                                                                                                                                                                                                                                                                                                                                                                                                                                                                                                                                                                                                                                                                                                                                                                                                                                                                                                                                                   (16015523*cos(t5))/40000000000 - (713241*sin(t5)*sin(t6))/100000000000 - (817*d5*cos(t5)*cos(t6))/2000000 + (817*d6*sin(t5)*sin(t6))/2000000;
                                                                                                                                                                                                                                                                                                                                                                                                                                                                                                                                                                                                                                                                                                                                                                                                                                                                                                                                                                                                                                                                                                                                                                                                                                         (713241*cos(t2 + t3 + t4 + t5 + t6))/400000000000 + (33478847947*cos(t2 + t3 + t4))/10000000000000 + (713241*cos(t2 + t3 + t4 + t5 - t6))/400000000000 - (713241*cos(t2 + t3 + t4 - t5 + t6))/400000000000 - (784477*cos(t2 + t3 + t4 + t5 - 2*t6))/320000000000 + (784477*cos(t2 + t3 + t4 + t5 + 2*t6))/320000000000 - (49450651*cos(t2 + t3 + t4 + t5))/250000000000 - (713241*cos(t2 + t3 + t4 - t5 - t6))/400000000000 - (784477*cos(t2 + t3 + t4 - t5 - 2*t6))/320000000000 + (784477*cos(t2 + t3 + t4 - t5 + 2*t6))/320000000000 + (49450651*cos(t2 + t3 + t4 - t5))/250000000000 + (784477*cos(t2 + t3 + t4 - 2*t6))/160000000000 + (784477*cos(t2 + t3 + t4 + 2*t6))/160000000000 - (817*a3*sin(t2 + t3 - t5 - t6))/8000000 - (817*d4*cos(t2 + t3 + t4 + t5 - t6))/8000000 - (817*d4*cos(t2 + t3 + t4 - t5 + t6))/8000000 - (817*d5*cos(t2 + t3 + t4 + t5 - t6))/8000000 + (817*d5*cos(t2 + t3 + t4 - t5 + t6))/8000000 - (817*d6*cos(t2 + t3 + t4 + t5 - t6))/8000000 + (817*d6*cos(t2 + t3 + t4 - t5 + t6))/8000000 + (43*d6^2*cos(t2 + t3 + t4))/100 - (582539*a3*sin(t2 + t3 - t5))/100000000 - (817*a2*sin(t2 + t5 - t6))/8000000 + (817*a2*sin(t2 - t5 + t6))/8000000 + (817*a2*sin(t5 - t2 + t6))/8000000 + (582539*d4*cos(t2 + t3 + t4 + t5))/100000000 + (582539*d5*cos(t2 + t3 + t4 + t5))/100000000 + (817*a3*sin(t2 + t3 + t5 + t6))/8000000 + (582539*a2*sin(t2 + t5))/100000000 + (817*d4*cos(t2 + t3 + t4 - t5 - t6))/8000000 - (817*d5*cos(t2 + t3 + t4 - t5 - t6))/8000000 + (817*d6*cos(t2 + t3 + t4 - t5 - t6))/8000000 + (582539*d4*cos(t2 + t3 + t4 - t5))/100000000 - (582539*d5*cos(t2 + t3 + t4 - t5))/100000000 - (817*a3*sin(t2 + t3 + t5 - t6))/8000000 + (817*a3*sin(t2 + t3 - t5 + t6))/8000000 + (817*d4*cos(t2 + t3 + t4 + t5 + t6))/8000000 + (817*d5*cos(t2 + t3 + t4 + t5 + t6))/8000000 - (817*d6*cos(t2 + t3 + t4 + t5 + t6))/8000000 - (582539*a2*sin(t2 - t5))/100000000 - (37539*d6*cos(t2 + t3 + t4))/2500000 + (582539*a3*sin(t2 + t3 + t5))/100000000 + (817*a2*sin(t2 + t5 + t6))/8000000 + (43*d4*d6*cos(t2 + t3 + t4 - t5))/200 - (43*d5*d6*cos(t2 + t3 + t4 - t5))/200 - (43*a2*d6*sin(t2 - t5))/200 + (43*a3*d6*sin(t2 + t3 + t5))/200 - (43*a3*d6*sin(t2 + t3 - t5))/200 + (43*d4*d6*cos(t2 + t3 + t4 + t5))/200 + (43*d5*d6*cos(t2 + t3 + t4 + t5))/200 + (43*a2*d6*sin(t2 + t5))/200,                                                                                                                                                                                                                                                                                                                                                                                                                                                                                                                                                                                                                                                                                                                                                                                                                                                                                                                                                                                                                                                                                                                                                                                                                                                                                                                                                                                                                                                                                                                                                                                                                                                                                                                                                                                                                                                                                                                                                                                                                                                                                                                                                                                                                                                                                                                                                                                                                                                                                                                                                                                                                                                                                                                                                                                                              (49450651*cos(t5))/125000000000 - (713241*cos(t5)*cos(t6))/100000000000 - (582539*d5*cos(t5))/50000000 + (784477*cos(t6)*sin(t5)*sin(t6))/40000000000 + (817*d6*cos(t5)*cos(t6))/2000000 + (582539*a3*cos(t5)*sin(t4))/50000000 + (817*d5*sin(t5)*sin(t6))/2000000 - (43*d5*d6*cos(t5))/100 + (582539*a2*cos(t3)*cos(t5)*sin(t4))/50000000 + (582539*a2*cos(t4)*cos(t5)*sin(t3))/50000000 - (817*a3*sin(t4)*sin(t5)*sin(t6))/2000000 + (43*a3*d6*cos(t5)*sin(t4))/100 - (817*a2*cos(t3)*sin(t4)*sin(t5)*sin(t6))/2000000 - (817*a2*cos(t4)*sin(t3)*sin(t5)*sin(t6))/2000000 + (43*a2*d6*cos(t3)*cos(t5)*sin(t4))/100 + (43*a2*d6*cos(t4)*cos(t5)*sin(t3))/100,                                                                                                                                                                                                                                                                                                                                                                                                                                                                                                                                                                                                                                                                                                                                                                                                                                                                                                                                                                                                                                                                                                                                                                                                                                                                                                                                                                                                                                                                                                                                                                                                                                                                                                                                                                                                                                                                                                                                                                                                                                                                                                                                                                                                                                                                                                                                                                                                                                                                                                                                                                                                                                                                                                                          (49450651*cos(t5))/125000000000 - (713241*cos(t5)*cos(t6))/100000000000 - (582539*d5*cos(t5))/50000000 + (784477*cos(t6)*sin(t5)*sin(t6))/40000000000 + (817*d6*cos(t5)*cos(t6))/2000000 + (582539*a3*cos(t5)*sin(t4))/50000000 + (817*d5*sin(t5)*sin(t6))/2000000 - (43*d5*d6*cos(t5))/100 - (817*a3*sin(t4)*sin(t5)*sin(t6))/2000000 + (43*a3*d6*cos(t5)*sin(t4))/100,                                                                                                                                                                                                                                                                                                                                                                                                                                                                                                                                                                                                                                                                                                                                                                                                                                                                                                                                                                                                                                                                                                                                                                                                                                                                                                                                                                                                                                                                                                                                                                                                                                                                                                                                                                                                                                                                                                                                                                                                                                                                                                                                                                                                                                                                                                                                                                                                             (49450651*cos(t5))/125000000000 - (713241*cos(t5)*cos(t6))/100000000000 - (582539*d5*cos(t5))/50000000 + (784477*cos(t6)*sin(t5)*sin(t6))/40000000000 + (817*d6*cos(t5)*cos(t6))/2000000 + (817*d5*sin(t5)*sin(t6))/2000000 - (43*d5*d6*cos(t5))/100,                                                                                                                                                                                                                                                                                                                                                                                                                                                                                                                                                                                                                                                                                                                                                                                                                                                                                                                                                                                                                                                                                                                                                                                                                                                                                                                                                                                                                                                                                                                                                                                                                                                                                                                                                                                                                                                                                                                                                                                                                                                                                                                                                                                                                                                (43*d6^2)/100 - (37539*d6)/2500000 + (784477*cos(2*t6))/80000000000 + 33478847947/10000000000000,                                                                                                                                                                                                                                                                                                                                                                                                                                                                                                                                                                                                                                                                                                                                                                                                                                                                                                                                                                                                                                                                                                                                                                                                                                                                                                                                                                                                                                                                                                                                                                                                                                                                                                                                                                                                                                                                                                                                                                                                    (817*cos(t6)*(50000*d6 - 873))/100000000000;
                                                                                                                                                                                                                                                                                                                                                                                                                                                                                                                                                                                                                                                                                                                                                                                                                                                                                                                                                                                                                                                                                                                                                                                                                                                                                                                                                                                                                                                                                                                                          (817*a2*cos(t2)*cos(t6)*sin(t5))/2000000 - (713241*cos(t2)*cos(t3)*cos(t4)*cos(t6))/100000000000 + (16015523*cos(t2)*cos(t3)*sin(t4)*sin(t5))/40000000000 + (16015523*cos(t2)*cos(t4)*sin(t3)*sin(t5))/40000000000 + (16015523*cos(t3)*cos(t4)*sin(t2)*sin(t5))/40000000000 + (713241*cos(t2)*cos(t6)*sin(t3)*sin(t4))/100000000000 + (713241*cos(t3)*cos(t6)*sin(t2)*sin(t4))/100000000000 + (713241*cos(t4)*cos(t6)*sin(t2)*sin(t3))/100000000000 - (16015523*sin(t2)*sin(t3)*sin(t4)*sin(t5))/40000000000 + (817*d6*cos(t2)*cos(t3)*cos(t4)*cos(t6))/2000000 + (817*a3*cos(t2)*cos(t3)*cos(t6)*sin(t5))/2000000 - (817*d4*cos(t2)*cos(t3)*sin(t4)*sin(t6))/2000000 - (817*d4*cos(t2)*cos(t4)*sin(t3)*sin(t6))/2000000 - (817*d4*cos(t3)*cos(t4)*sin(t2)*sin(t6))/2000000 - (817*d6*cos(t2)*cos(t6)*sin(t3)*sin(t4))/2000000 - (817*d6*cos(t3)*cos(t6)*sin(t2)*sin(t4))/2000000 - (817*d6*cos(t4)*cos(t6)*sin(t2)*sin(t3))/2000000 - (817*a3*cos(t6)*sin(t2)*sin(t3)*sin(t5))/2000000 + (817*d4*sin(t2)*sin(t3)*sin(t4)*sin(t6))/2000000 + (713241*cos(t2)*cos(t3)*cos(t5)*sin(t4)*sin(t6))/100000000000 + (713241*cos(t2)*cos(t4)*cos(t5)*sin(t3)*sin(t6))/100000000000 + (713241*cos(t3)*cos(t4)*cos(t5)*sin(t2)*sin(t6))/100000000000 - (713241*cos(t5)*sin(t2)*sin(t3)*sin(t4)*sin(t6))/100000000000 - (817*d4*cos(t2)*cos(t5)*cos(t6)*sin(t3)*sin(t4))/2000000 - (817*d4*cos(t3)*cos(t5)*cos(t6)*sin(t2)*sin(t4))/2000000 - (817*d4*cos(t4)*cos(t5)*cos(t6)*sin(t2)*sin(t3))/2000000 - (817*d5*cos(t2)*cos(t3)*cos(t6)*sin(t4)*sin(t5))/2000000 - (817*d5*cos(t2)*cos(t4)*cos(t6)*sin(t3)*sin(t5))/2000000 - (817*d5*cos(t3)*cos(t4)*cos(t6)*sin(t2)*sin(t5))/2000000 - (817*d6*cos(t2)*cos(t3)*cos(t5)*sin(t4)*sin(t6))/2000000 - (817*d6*cos(t2)*cos(t4)*cos(t5)*sin(t3)*sin(t6))/2000000 - (817*d6*cos(t3)*cos(t4)*cos(t5)*sin(t2)*sin(t6))/2000000 + (817*d5*cos(t6)*sin(t2)*sin(t3)*sin(t4)*sin(t5))/2000000 + (817*d6*cos(t5)*sin(t2)*sin(t3)*sin(t4)*sin(t6))/2000000 + (817*d4*cos(t2)*cos(t3)*cos(t4)*cos(t5)*cos(t6))/2000000,                                                                                                                                                                                                                                                                                                                                                                                                                                                                                                                                                                                                                                                                                                                                                                                                                                                                                                                                                                                                                                                                                                                                                                                                                                                                                                                                                                                                                                                                                                                                                                                                                                                                                                                                                                                                                                                                                                                                                                                                                                                                                                                                                                                                                                                                                                                                                                                                                                                                                                                                                                                                                                                                                                                                                                                                                                                                                                                                                                                                                                                     (16015523*cos(t5))/40000000000 - (713241*sin(t5)*sin(t6))/100000000000 - (817*d5*cos(t5)*cos(t6))/2000000 + (817*a3*cos(t4)*sin(t6))/2000000 + (817*d6*sin(t5)*sin(t6))/2000000 + (817*a2*cos(t3)*cos(t4)*sin(t6))/2000000 + (817*a3*cos(t5)*cos(t6)*sin(t4))/2000000 - (817*a2*sin(t3)*sin(t4)*sin(t6))/2000000 + (817*a2*cos(t3)*cos(t5)*cos(t6)*sin(t4))/2000000 + (817*a2*cos(t4)*cos(t5)*cos(t6)*sin(t3))/2000000,                                                                                                                                                                                                                                                                                                                                                                                                                                                                                                                                                                                                                                                                                                                                                                                                                                                                                                                                                                                                                                                                                                                                                                                                                                                                                                                                                                                                                                                                                                                                                                                                                                                                                                                                                                                                                                                                                                                                                                                                                                                                                                                                                                                                                                                                                                                                                                                                                                                                                                                                                                                                                                                                                                                                                                                                                                                                       (16015523*cos(t5))/40000000000 - (713241*sin(t5)*sin(t6))/100000000000 - (817*d5*cos(t5)*cos(t6))/2000000 + (817*a3*cos(t4)*sin(t6))/2000000 + (817*d6*sin(t5)*sin(t6))/2000000 + (817*a3*cos(t5)*cos(t6)*sin(t4))/2000000,                                                                                                                                                                                                                                                                                                                                                                                                                                                                                                                                                                                                                                                                                                                                                                                                                                                                                                                                                                                                                                                                                                                                                                                                                                                                                                                                                                                                                                                                                                                                                                                                                                                                                                                                                                                                                                                                                                                                                                                                                                                                                                                                                                                                                                                                                                                                                                                                                                                                                                                     (16015523*cos(t5))/40000000000 - (713241*sin(t5)*sin(t6))/100000000000 - (817*d5*cos(t5)*cos(t6))/2000000 + (817*d6*sin(t5)*sin(t6))/2000000,                                                                                                                                                                                                                                                                                                                                                                                                                                                                                                                                                                                                                                                                                                                                                                                                                                                                                                                                                                                                                                                                                                                                                                                                                                                                                                                                                                                                                                                                                                                                                                                                                                                                                                                                                                                                                                                                                                                                                                                                                                                                                                                                                                                                                                                                                                     (817*cos(t6)*(50000*d6 - 873))/100000000000,                                                                                                                                                                                                                                                                                                                                                                                                                                                                                                                                                                                                                                                                                                                                                                                                                                                                                                                                                                                                                                                                                                                                                                                                                                                                                                                                                                                                                                                                                                                                                                                                                                                                                                                                                                                                                                                                                                                                                                                                                           16015523/40000000000];
 
end
